simulink subsystem "drone_model"  (R2023a)
settings: Solver=VariableStepAuto  StartTime=0.0  StopTime=10.0  RelTol=1e-3
undefined symbols (not defined in the file): C_D_drone, G_radu, k_loss, kF, kM, param, S_x, S_y, S_z
libraries: shared6dof x1, aerolibatmos2 x1
settings Model: Creator=timme  LastModifiedBy=raduserseniuc

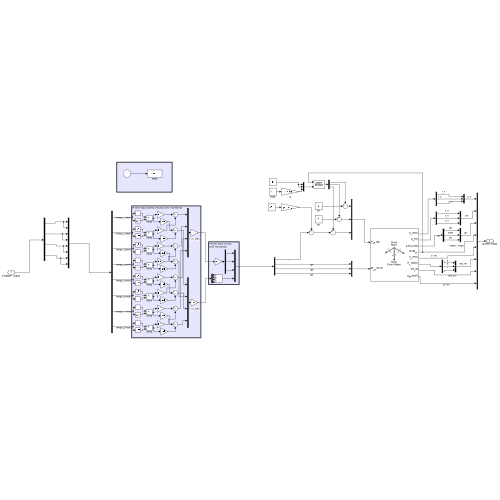
[thumbnail: Simulink's stored preview of the top-level diagram]
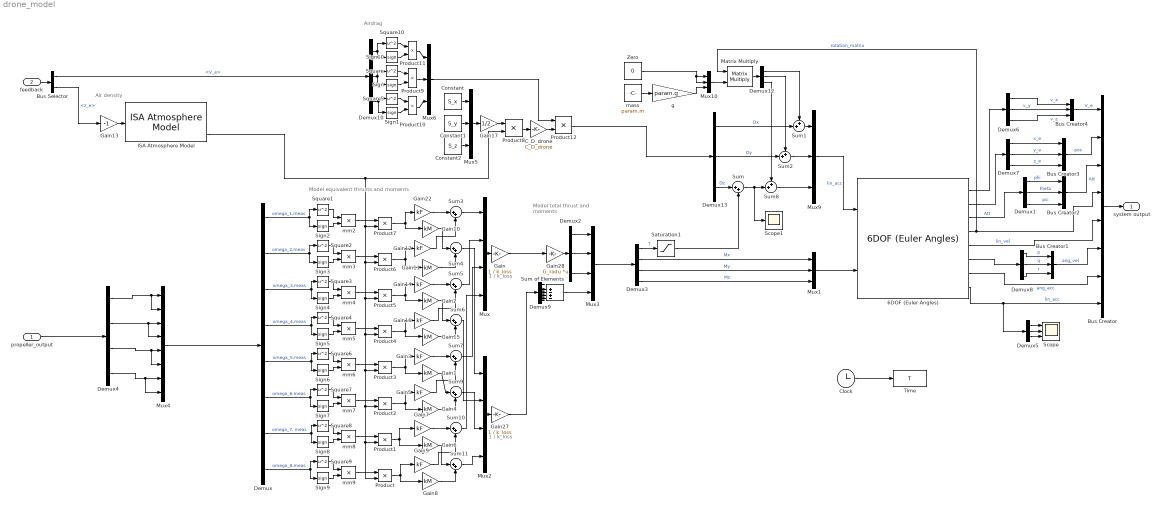
== system drone_model ==
  note: Airdrag
  note: Air density
  note: Model total thrust
      | and moments
  note: 1 / k_loss
  note: Model equivalent thrusts and moments
  note: 1 / k_loss
  propeller_output : Inport
  feedback : Inport  Port=2
  6DOF (Euler Angles) : shared6dof/6DOF (Euler Angles)  units=Metric (MKS)  mtype=Fixed  rep=Euler Angles  xme_0=[0 0 0]  Vm_0=[0 0 0]  eul_0=[0 0 0]  pm_0=[0 0 0]  mass_0=param.m  mass_e=0.5  mass_f=2.0  inertia=param.I  inertia_e=eye(3)  inertia_f=2*eye(3)  k_quat=1.0  vre_flag=on  abi_flag=off  aMode=0  xme_statename=''  Vm_statename=''  eul_statename=''  quat_statename=''  pm_statename=''  mass_statename=''
  Bus Creator : BusCreator  Inputs=8
  Bus Creator{1..4} (4 alike) : BusCreator  Inputs=3
  Bus Selector : BusSelector  OutputSignals=V_e,pos.z_e
  C_D_drone : Gain  Gain=C_D_drone
  Clock : Clock
  Constant : Constant  Value=S_x
  Constant1 : Constant  Value=S_y
  Constant2 : Constant  Value=S_z
  Demux : Demux  Outputs=8
  Demux{1..2,5..8,10,12..13} (9 alike) : Demux  Outputs=3
  Demux3 : Demux
  Demux4 : Demux
  Demux9 : Demux
  Gain : Gain  Gain=1 / k_loss
  Gain{1..2,4,6,8,10..11,15} (8 alike) : Gain  Gain=kM
  Gain{3,5,7,9,12,14,16,22} (8 alike) : Gain  Gain=kF
  Gain13 : Gain  Gain=-1
  Gain17 : Gain  Gain=1/2
  Gain27 : Gain  Gain=1 / k_loss
  Gain28 : Gain  Gain=G_radu  Multiplication=Matrix(K*u)
  ISA Atmosphere Model : aerolibatmos2/ISA Atmosphere Model  custom=off  g=9.80665  gamma=1.4  R=287.0531  L=0.0065  h_trop=11000  h_strat=20000  rho0=1.225  P0=101325  T0=288.15  h0=0
  Matrix Multiply : Product  Inputs=**  Multiplication=Matrix(*)
  Mux : Mux
  Mux{1,5..6,9..10} (5 alike) : Mux  Inputs=3
  Mux2 : Mux
  Mux3 : Mux
  Mux4 : Mux  Inputs=8
  Product{,1..12} (13 alike) : Product
  Saturation1 : Saturate  UpperLimit=200  LowerLimit=-200
  Scope : Scope  NumInputPorts=3
  Scope1 : Scope
  Sign{,1..10} (11 alike) : Signum
  Square{,1..10} (11 alike) : Math  Operator=square
  Sum{,3..7,9..11} (9 alike) : Sum  Inputs=|++
  Sum of Elements : Sum  Inputs=+|-|+|-
  Sum1 : Sum  Inputs=++|
  Sum2 : Sum  Inputs=++|
  Sum8 : Sum  Inputs=++|
  Time : ToWorkspace  VariableName=T  SampleTime=-1
      settings: Decimation=100
  Zero : Constant  Value=0  OutDataTypeStr=Inherit: Inherit via back propagation
  g : Gain  Gain=param.g
  mass : Constant  Value=param.m
  mm{2..9} (8 alike) : Product
  system output : Outport
  wires:
  Clock/1 -> Time/1
  6DOF (Euler Angles)/2 -> Demux7/1
  Mux1/1 -> 6DOF (Euler Angles)/2
  6DOF (Euler Angles)/7 -> Bus Creator/7  "ang_acc"
  6DOF (Euler Angles)/4 -> Bus Creator/4, Matrix Multiply/1  "rotation_matrix"
  6DOF (Euler Angles)/1 -> Demux6/1
  6DOF (Euler Angles)/5 -> Bus Creator/5  "lin_vel"
  6DOF (Euler Angles)/6 -> Demux8/1
  6DOF (Euler Angles)/3 -> Demux1/1  "Att"
  Bus Creator/1 -> system output/1
  Demux8/3 -> Bus Creator1/3  "r"
  Demux8/2 -> Bus Creator1/2  "q"
  Demux8/1 -> Bus Creator1/1  "p"
  Demux1/3 -> Bus Creator2/3  "psi"
  Demux1/2 -> Bus Creator2/2  "theta"
  Demux1/1 -> Bus Creator2/1  "phi"
  Demux7/3 -> Bus Creator3/3  "z_e"
  Demux7/2 -> Bus Creator3/2  "y_e"
  Demux7/1 -> Bus Creator3/1  "x_e"
  Demux6/3 -> Bus Creator4/3  "v_z"
  Demux6/2 -> Bus Creator4/2  "v_y"
  Demux6/1 -> Bus Creator4/1  "v_x"
  Bus Creator4/1 -> Bus Creator/1  "V_e"
  Bus Creator1/1 -> Bus Creator/6  "ang_vel"
  Bus Creator2/1 -> Bus Creator/3  "Att"
  Bus Creator3/1 -> Bus Creator/2  "pos"
  g/1 -> Mux10/3
  Mux10/1 -> Matrix Multiply/2
  Demux13/1 -> Sum1/2  "Dx"
  Demux12/3 -> Sum8/1
  Demux12/2 -> Sum2/1
  Sum2/1 -> Mux9/2
  mass/1 -> g/1
  Demux12/1 -> Sum1/1
  Zero/1 -> Mux10/2, Mux10/1
  Sum1/1 -> Mux9/1
  Sum8/1 -> Mux9/3
  Matrix Multiply/1 -> Demux12/1
  Demux13/2 -> Sum2/2  "Dy"
  Product7/1 -> Gain10/1, Gain22/1
  Gain12/1 -> Sum3/2
  Gain22/1 -> Sum3/1
  Product6/1 -> Gain11/1, Gain12/1
  Gain10/1 -> Sum4/1
  Product5/1 -> Gain2/1, Gain14/1
  Gain11/1 -> Sum4/2
  Product4/1 -> Gain15/1, Gain16/1
  Sign2/1 -> mm2/2
  Square1/1 -> mm2/1
  Square2/1 -> mm3/1
  Sign3/1 -> mm3/2
  Square3/1 -> mm4/1
  Sign4/1 -> mm4/2
  Square4/1 -> mm5/1
  Sign5/1 -> mm5/2
  Demux/1 -> Sign2/1, Square1/1  "omega_1,meas"
  Demux/2 -> Sign3/1, Square2/1  "omega_2,meas"
  Demux/3 -> Sign4/1, Square3/1  "omega_3,meas"
  Demux/4 -> Sign5/1, Square4/1  "omega_4,meas"
  Demux3/2 -> Mux1/1  "Mx"
  Demux3/3 -> Mux1/2  "My"
  Demux3/4 -> Mux1/3  "Mz"
  Demux3/1 -> Saturation1/1  "T"
  Sign6/1 -> mm6/2
  Product3/1 -> Gain1/1, Gain3/1
  Square6/1 -> mm6/1
  Demux/5 -> Sign6/1, Square6/1  "omega_5,meas"
  Product2/1 -> Gain5/1, Gain4/1
  Sign7/1 -> mm7/2
  Square7/1 -> mm7/1
  Demux/6 -> Square7/1, Sign7/1  "omega_6,meas"
  Sign8/1 -> mm8/2
  Square8/1 -> mm8/1
  mm9/1 -> Product/1
  Sign9/1 -> mm9/2
  Square9/1 -> mm9/1
  Demux/7 -> Sign8/1, Square8/1  "omega_7, meas"
  Demux/8 -> Sign9/1, Square9/1  "omega_8,meas"
  Gain16/1 -> Sum5/2
  Gain14/1 -> Sum5/1
  Gain15/1 -> Sum6/2
  Gain2/1 -> Sum6/1
  Gain3/1 -> Sum7/1
  Gain4/1 -> Sum9/2
  Gain1/1 -> Sum9/1
  Gain5/1 -> Sum7/2
  Gain9/1 -> Sum10/2
  Gain7/1 -> Sum10/1
  Gain8/1 -> Sum11/2
  Gain6/1 -> Sum11/1
  Sum3/1 -> Mux/1
  Sum5/1 -> Mux/2
  Sum7/1 -> Mux/3
  Sum10/1 -> Mux/4
  Sum11/1 -> Mux2/4
  Sum9/1 -> Mux2/3
  Sum6/1 -> Mux2/2
  Sum4/1 -> Mux2/1
  Mux/1 -> Gain/1
  Mux2/1 -> Gain27/1
  Gain/1 -> Gain28/1
  Sum of Elements/1 -> Mux3/4
  Gain28/1 -> Demux2/1
  Demux2/3 -> Mux3/3
  Demux2/2 -> Mux3/2
  Demux2/1 -> Mux3/1
  Mux3/1 -> Demux3/1
  Demux9/1 -> Sum of Elements/1
  Demux9/2 -> Sum of Elements/2
  Demux9/3 -> Sum of Elements/3
  Demux9/4 -> Sum of Elements/4
  Gain27/1 -> Demux9/1
  Demux4/1 -> Mux4/2, Mux4/1
  Demux4/2 -> Mux4/4, Mux4/3
  Demux4/3 -> Mux4/6, Mux4/5
  Demux4/4 -> Mux4/8, Mux4/7
  propeller_output/1 -> Demux4/1
  Mux4/1 -> Demux/1
  Mux9/1 -> 6DOF (Euler Angles)/1  "lin_acc"
  6DOF (Euler Angles)/8 -> Bus Creator/8, Demux5/1  "lin_acc"
  Demux5/2 -> Scope/2
  Demux5/1 -> Scope/1
  Demux5/3 -> Scope/3
  Sum/1 -> Sum8/2, Scope1/1
  feedback/1 -> Bus Selector/1
  Product/1 -> Gain9/1, Gain8/1
  mm8/1 -> Product1/1
  Product1/1 -> Gain7/1, Gain6/1
  mm7/1 -> Product2/1
  mm6/1 -> Product3/1
  mm5/1 -> Product4/1
  mm4/1 -> Product5/1
  mm3/1 -> Product6/1
  mm2/1 -> Product7/1
  Gain13/1 -> ISA Atmosphere Model/1
  Constant/1 -> Mux5/1
  Constant1/1 -> Mux5/2
  Constant2/1 -> Mux5/3
  Mux5/1 -> Gain17/1
  Gain17/1 -> Product8/1
  ISA Atmosphere Model/4 -> Product8/2, Product7/2, Product6/2, Product5/2, Product4/2, Product3/2, Product2/2, Product1/2, Product/2
  Square/1 -> Product9/1
  Sign/1 -> Product9/2
  Sign1/1 -> Product10/2
  Square5/1 -> Product10/1
  Sign10/1 -> Product11/2
  Square10/1 -> Product11/1
  Demux10/1 -> Sign10/1, Square10/1
  Demux10/2 -> Sign/1, Square/1
  Demux10/3 -> Sign1/1, Square5/1
  Product8/1 -> C_D_drone/1
  C_D_drone/1 -> Product12/2
  Product10/1 -> Mux6/3
  Product9/1 -> Mux6/2
  Product11/1 -> Mux6/1
  Mux6/1 -> Product12/1
  Bus Selector/2 -> Gain13/1  "<z_e>"
  Saturation1/1 -> Sum/2
  Demux13/3 -> Sum/1  "Dz"
  Product12/1 -> Demux13/1
  Bus Selector/1 -> Demux10/1  "<V_e>"
